simulink model "math_operation"  (R2019b)
settings: Solver=VariableStepAuto  StartTime=0.0  StopTime=10.0  RelTol=1e-3
libraries: simulink x2
settings Model: Creator=46769  LastModifiedBy=chiragg
settings DebuggingCC: SFMachineParentedDataDiag=error

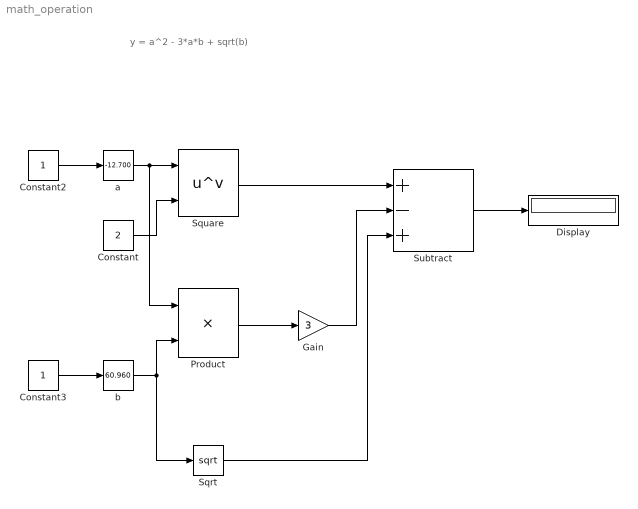
== system math_operation ==
  note: y = a^2 - 3*a*b + sqrt(b)
  Constant : Constant  Value=2
  Constant2 : Constant
  Constant3 : Constant
  Display : Display
  Gain : Gain  Gain=3
  Product : Product
  Sqrt : Sqrt  SaturateOnIntegerOverflow=on
  Square : Math  Operator=pow  SignedPower=off  SaturateOnIntegerOverflow=on
  Subtract : Sum  Inputs=+-+
  a : simulink/Math Operations/Slider Gain  gain=-12.700  low=-127  high=127
  b : simulink/Math Operations/Slider Gain  gain=60.960  low=-127  high=127
  wires:
  Constant2/1 -> a/1
  Constant3/1 -> b/1
  a/1 -> Product/1, Square/1
  Constant/1 -> Square/2
  b/1 -> Sqrt/1, Product/2
  Square/1 -> Subtract/1
  Product/1 -> Gain/1
  Gain/1 -> Subtract/2
  Sqrt/1 -> Subtract/3
  Subtract/1 -> Display/1
